simulink model "second"  (R2024b)
settings: Solver=VariableStepAuto  StartTime=0.0  StopTime=45  RelTol=1e-3
settings Model: Creator=asus  LastModifiedBy=asus
settings HardwareCC: TargetBitPerPointer=64  TargetBitPerSizeT=64  TargetBitPerPtrDiffT=64  TargetLongLongMode=on  TargetIntDivRoundTo=Zero  TargetEndianess=LittleEndian  TargetWordSize=64  TargetHWDeviceType=MATLAB Host  ProdEqTarget=off
settings RTWCC: Description=Rapid Simulation Target  SystemTargetFile=rsim.tlc  TemplateMakefile=rsim_default_tmf
settings RSimTargetCC: TargetLangStandard=C99 (ISO)  InstructionSetFMA=off  OptimizeReductions=off  LogToMDFFile=off

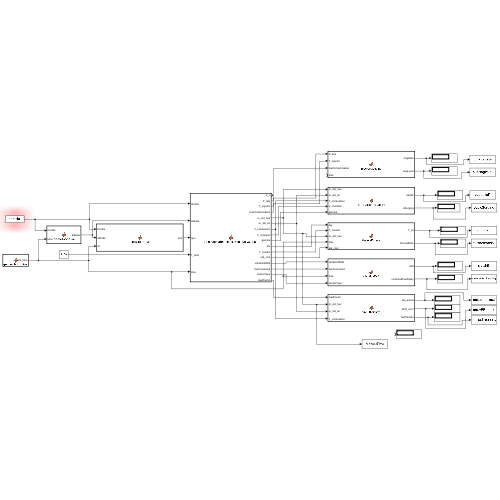
[thumbnail: Simulink's stored preview of the top-level diagram]
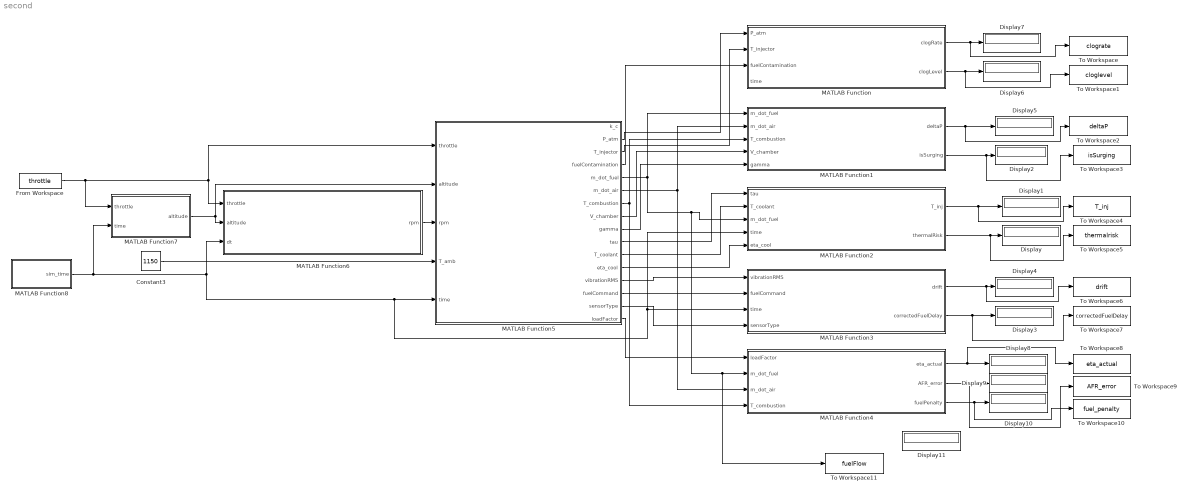
== system second ==
  Constant3 : Constant  Value=1150
  Display{,1..11} (12 alike) : Display
  From Workspace : FromWorkspace  VariableName=throttle
  MATLAB Function : MATLAB Function  TreatAsAtomicUnit=on
  MATLAB Function1 : MATLAB Function  TreatAsAtomicUnit=on
  MATLAB Function2 : MATLAB Function  TreatAsAtomicUnit=on
  MATLAB Function3 : MATLAB Function  TreatAsAtomicUnit=on
  MATLAB Function4 : MATLAB Function  TreatAsAtomicUnit=on
  MATLAB Function5 : MATLAB Function  TreatAsAtomicUnit=on
  MATLAB Function6 : MATLAB Function  TreatAsAtomicUnit=on
  MATLAB Function7 : MATLAB Function  TreatAsAtomicUnit=on
  MATLAB Function8 : MATLAB Function  TreatAsAtomicUnit=on
  To Workspace : ToWorkspace  VariableName=clograte  SaveFormat=Timeseries  SampleTime=-1
  To Workspace1 : ToWorkspace  VariableName=cloglevel  SaveFormat=Timeseries  SampleTime=-1
  To Workspace10 : ToWorkspace  VariableName=fuel_penalty  SaveFormat=Timeseries  SampleTime=-1
  To Workspace11 : ToWorkspace  VariableName=fuelFlow  SaveFormat=Timeseries  SampleTime=-1
  To Workspace2 : ToWorkspace  VariableName=deltaP  SaveFormat=Timeseries  SampleTime=-1
  To Workspace3 : ToWorkspace  VariableName=isSurging  SaveFormat=Timeseries  SampleTime=-1
  To Workspace4 : ToWorkspace  VariableName=T_inj  SaveFormat=Timeseries  SampleTime=-1
  To Workspace5 : ToWorkspace  VariableName=thermalrisk  SaveFormat=Timeseries  SampleTime=-1
  To Workspace6 : ToWorkspace  VariableName=drift  SaveFormat=Timeseries  SampleTime=-1
  To Workspace7 : ToWorkspace  VariableName=correctedFuelDelay  SaveFormat=Timeseries  SampleTime=-1
  To Workspace8 : ToWorkspace  VariableName=eta_actual  SaveFormat=Timeseries  SampleTime=-1
  To Workspace9 : ToWorkspace  VariableName=AFR_error  SaveFormat=Timeseries  SampleTime=-1
  wires:
  MATLAB Function6/1(rpm) -> MATLAB Function5/3(rpm)
  From Workspace/1 -> MATLAB Function6/1(throttle), MATLAB Function5/1(throttle), MATLAB Function7/1(throttle)
  MATLAB Function7/1(altitude) -> MATLAB Function5/2(altitude), MATLAB Function6/2(altitude)
  MATLAB Function8/1(sim_time) -> MATLAB Function7/2(time), MATLAB Function3/3(time), MATLAB Function2/4(time), MATLAB Function5/5(time), MATLAB Function6/3(dt)
  MATLAB Function5/4(fuelContamination) -> MATLAB Function/3(fuelContamination)
  MATLAB Function5/3(T_injector) -> MATLAB Function/2(T_injector)
  MATLAB Function5/2(P_atm) -> MATLAB Function/1(P_atm)
  MATLAB Function5/5(m_dot_fuel) -> MATLAB Function2/3(m_dot_fuel), To Workspace11/1, MATLAB Function4/2(m_dot_fuel), MATLAB Function1/1(m_dot_fuel)
  MATLAB Function5/6(m_dot_air) -> MATLAB Function4/3(m_dot_air), MATLAB Function1/2(m_dot_air)
  MATLAB Function5/7(T_combustion) -> MATLAB Function4/4(T_combustion), MATLAB Function1/3(T_combustion)
  MATLAB Function5/8(V_chamber) -> MATLAB Function1/4(V_chamber)
  MATLAB Function5/9(gamma) -> MATLAB Function1/5(gamma)
  MATLAB Function5/10(tau) -> MATLAB Function2/1(tau)
  MATLAB Function5/11(T_coolant) -> MATLAB Function2/2(T_coolant)
  MATLAB Function5/12(eta_cool) -> MATLAB Function2/5(eta_cool)
  MATLAB Function5/13(vibrationRMS) -> MATLAB Function3/1(vibrationRMS)
  MATLAB Function5/14(fuelCommand) -> MATLAB Function3/2(fuelCommand)
  MATLAB Function5/15(sensorType) -> MATLAB Function3/4(sensorType)
  MATLAB Function5/16(loadFactor) -> MATLAB Function4/1(loadFactor)
  Constant3/1 -> MATLAB Function5/4(T_amb)
  MATLAB Function2/2(thermalRisk) -> To Workspace5/1, Display/1
  MATLAB Function2/1(T_inj) -> To Workspace4/1, Display1/1
  MATLAB Function1/2(isSurging) -> To Workspace3/1, Display2/1
  MATLAB Function/1(clogRate) -> To Workspace/1, Display7/1
  MATLAB Function1/1(deltaP) -> To Workspace2/1, Display5/1
  MATLAB Function3/1(drift) -> To Workspace6/1, Display4/1
  MATLAB Function3/2(correctedFuelDelay) -> To Workspace7/1, Display3/1
  MATLAB Function4/2(AFR_error) -> To Workspace9/1, Display9/1
  MATLAB Function4/1(eta_actual) -> To Workspace8/1, Display8/1
  MATLAB Function4/3(fuelPenalty) -> To Workspace10/1, Display10/1
  MATLAB Function/2(clogLevel) -> To Workspace1/1, Display6/1

== matlab function second/MATLAB Function6 ==
  data: throttle input; rpm output; altitude input; dt input
function rpm = calculateRPM(throttle, altitude, dt)
    %#codegen
    
    % Input validation for Simulink and codegen
    coder.inline('always'); % Inline the function for efficiency
    assert(isscalar(throttle) && isreal(throttle) && throttle >= 0 && throttle <= 1, ...
           'Throttle must be a scalar in [0, 1]');
    assert(isscalar(altitude) && isreal(altitude) && altitude >= 0, ...
           'Altitude must be a non-negative scalar');
    assert(isscalar(dt) && isreal(dt) && dt > 0, ...
           'Time step (dt) must be a positive scalar');
    
    % Initialize persistent variable for RPM history
    persistent rpm_prev
    if isempty(rpm_prev)
        rpm_prev = 800.0; % Engine idle speed (double)
    end
    
    % Basic RPM calculation
    base_rpm = 800.0 + (throttle * 4000.0); % Linear throttle response (scaled for realistic RPM)
    altitude_factor = max(0.5, 1.0 - (altitude / 15000.0)); % Altitude compensation
    
    % Apply first-order lag to simulate engine response
    target_rpm = base_rpm * altitude_factor;
    time_constant = 2.0; % Seconds for 63% response
    rpm = rpm_prev + (target_rpm - rpm_prev) * (dt / time_constant);
    
    % Ensure RPM stays within realistic bounds
    rpm = min(max(rpm, 800.0), 6000.0); % Bound RPM between idle (800) and max (6000)
    
    % Store current RPM for next iteration
    rpm_prev = rpm;
    
    % Ensure output is scalar double
    rpm = double(rpm);
end

== matlab function second/MATLAB Function7 ==
  data: throttle input; altitude output; time input
function altitude = throttleToAltitude(throttle, time)
    % Constants
    max_thrust = 50000;   % N (adjust per helicopter)
    m = 3000;             % kg
    g = 9.81;             % m/s²
    k = 1.3;              % Drag factor
    
    % Thrust calculation
    T = (throttle/100) * max_thrust;
    
    % Vertical acceleration
    dh_dt = (T - m*g) / (m*k);
    
    % Integrate to get altitude
    persistent alt_prev;
    if isempty(alt_prev)
        alt_prev = 0;  % Start at ground level
    end
    altitude = alt_prev + dh_dt * time;
    altitude = max(0, altitude);  % No negative altitude
    alt_prev = altitude;
end

== matlab function second/MATLAB Function8 ==
  data: sim_time output
function sim_time = getSimulationTime()
    persistent start_time;
    if isempty(start_time)
        start_time = posixtime(datetime('now'));  % Unix timestamp at start
    end
    sim_time = posixtime(datetime('now')) - start_time;  % Elapsed seconds
end

== matlab function second/MATLAB Function1 ==
  data: m_dot_fuel input; deltaP output; m_dot_air input; T_combustion input; V_chamber input; isSurging output; gamma input
function [deltaP, isSurging] = combustionInstability(m_dot_fuel, m_dot_air, T_combustion, V_chamber, gamma)
    % Inputs:
    %   m_dot_fuel (kg/s): Fuel mass flow rate
    %   m_dot_air (kg/s): Air mass flow rate
    %   T_combustion (K): Combustion temperature
    %   V_chamber (m³): Combustion chamber volume
    %   gamma: Specific heat ratio (e.g., 1.4 for air)
    
    % Constants
    R = 287;  % Gas constant for air (J/kg·K)
    surgeThreshold = 0.3;  % Threshold for surge detection (empirical)
    
    % Pressure oscillation amplitude (simplified model)
    FAR_actual = m_dot_fuel / m_dot_air;
    FAR_stoich = 0.068;  % Stoichiometric FAR for kerosene-air
    deltaP = sqrt(gamma * R * T_combustion / V_chamber) * abs(FAR_actual - FAR_stoich);
    
    % Surging detection (boolean)
    isSurging = (deltaP > surgeThreshold);
end

== matlab function second/MATLAB Function ==
  data: P_atm input; clogRate output; T_injector input; fuelContamination input; time input; clogLevel output
function [clogRate, clogLevel] = injectorClogging(P_atm, T_injector, fuelContamination, time)
    % Inputs:
    %   P_atm (Pa): Ambient pressure (altitude-dependent)
    %   T_injector (K): Injector temperature
    %   fuelContamination (0-1): Fuel impurity level
    %   time (s): Simulation time (for integration)
    
    % Constants
    P_ref = 101325;     % Reference pressure (Pa, sea level)
    R = 8.314;          % Universal gas constant
    E_a = 50000;        % Activation energy (J/mol, empirical)
    k_c = 0.001;        % Empirical clogging rate constant
    
    % Clogging rate (dC/dt)
    clogRate = k_c * (P_atm / P_ref) * exp(-E_a / (R * T_injector)) * fuelContamination;
    
    % Clog level (integrate rate over time)
    persistent cumulativeClog;
    if isempty(cumulativeClog)
        cumulativeClog = 0;
    end
    cumulativeClog = cumulativeClog + clogRate * time;
    clogLevel = min(cumulativeClog, 100);  % Cap at 100%
end

== matlab function second/MATLAB Function2 ==
  data: tau input; T_coolant input; m_dot_fuel input; T_inj output; time input; thermalRisk output; eta_cool input
function [T_inj, thermalRisk] = thermalStress(tau, T_coolant, m_dot_fuel, time, eta_cool)
    %#codegen
    % Constants
    T_max = 500;          % Max allowable injector temp (K)
    k_heat = 0.05;        % Heat gain coefficient
    k_cool = 0.1;         % Cooling coefficient
    
    % 1. Heat generation (always >= 0)
    Q_gen = max(0, k_heat * abs(tau) * abs(m_dot_fuel));
    
    % 2. Heat dissipation (always >= 0)
    Q_cool = max(0, k_cool * abs(eta_cool) * (T_coolant - 298));
    
    % 3. Temperature calculation (Euler integration)
    persistent T_inj_prev;
    if isempty(T_inj_prev)
        T_inj_prev = T_coolant;  % Initialize to coolant temp
    end
    T_inj = T_inj_prev + (Q_gen - Q_cool) * time;
    T_inj = max(T_coolant, T_inj);  % Never below coolant temp
    T_inj_prev = T_inj;
    
    % 4. Non-negative thermal risk (0-1 scale)
    thermalRisk = max(0, min(1, (T_inj - 0.7*T_max)/(0.3*T_max)));
end

== matlab function second/MATLAB Function3 ==
  data: vibrationRMS input; fuelCommand input; time input; sensorType input; drift output; correctedFuelDelay output
function [drift, correctedFuelDelay] = vibrationDrift(vibrationRMS, fuelCommand, time, sensorType)
    % Inputs:
    %   vibrationRMS (m/s²): Vibration magnitude (RMS)
    %   fuelCommand (kg/s): Commanded fuel flow rate
    %   time (s): Simulation time
    %   sensorType: 1=Pressure, 2=Temperature (different drift behaviors)
    
    % Constants
    kBias = 0.02;       % Drift coefficient (empirical)
    kPhase = 1e-4;      % Phase delay coefficient
    maxDrift = 0.15;    % 15% max error
    
    % 1. Sensor Bias Drift (DC offset)
    drift = kBias * vibrationRMS * time;
    drift = min(drift, maxDrift);  % Clamp drift
    
    % 2. Fuel Delivery Delay (phase lag)
    if sensorType == 1
        % Pressure sensor: Delay ~ vibration^2
        phaseLag = kPhase * (vibrationRMS^2) * fuelCommand;
    else
        % Temperature sensor: Delay ~ linear
        phaseLag = kPhase * vibrationRMS * fuelCommand;
    end
    
    % Compensated delay (example: subtract estimated lag)
    correctedFuelDelay = max(0, fuelCommand - phaseLag);
end

== matlab function second/MATLAB Function4 ==
  data: loadFactor input; m_dot_fuel input; m_dot_air input; T_combustion input; eta_actual output; AFR_error output; fuelPenalty output
function [eta_actual, AFR_error, fuelPenalty] = fuelEfficiency(loadFactor, m_dot_fuel, m_dot_air, T_combustion)
    % Inputs:
    %   loadFactor (0-1): Current load / Rated load
    %   m_dot_fuel (kg/s): Fuel mass flow rate
    %   m_dot_air (kg/s): Air mass flow rate
    %   T_combustion (K): Combustion chamber temperature
    
    % Constants
    AFR_stoich = 14.7;       % Stoichiometric AFR for kerosene
    AFR_opt_map = [12.5, 14.7, 16.3];  % Optimal AFR at [0.3, 0.7, 1.0] loadFactor
    
    % 1. Interpolate optimal AFR for current load
    loadPoints = [0.3, 0.7, 1.0];
    AFR_opt = interp1(loadPoints, AFR_opt_map, loadFactor, 'pchip');
    
    % 2. Calculate actual AFR and error
    AFR_actual = m_dot_air / max(m_dot_fuel, 1e-6);  % Avoid division by zero
    AFR_error = AFR_actual - AFR_opt;
    
    % 3. Efficiency penalty (0-1 scale)
    T_norm = T_combustion / 1000;  % Normalized temperature
    fuelPenalty = exp(-0.5 * (AFR_error^2)) * (1 - 0.2 * loadFactor * T_norm);
    eta_actual = 0.95 * fuelPenalty;  % Baseline 95% efficiency scaled by penalty
end

== matlab function second/MATLAB Function5 ==
  data: throttle input; k_c output; altitude input; rpm input; T_amb input; P_atm output; time input; T_injector output; fuelContamination output; m_dot_fuel output; m_dot_air output; T_combustion output; V_chamber output; gamma output; tau output; T_coolant output; eta_cool output; vibrationRMS output; fuelCommand output; sensorType output; loadFactor output
function [k_c, P_atm, T_injector, fuelContamination, ...
          m_dot_fuel, m_dot_air, T_combustion, V_chamber, gamma, ...
          tau, T_coolant, eta_cool, ...
          vibrationRMS, fuelCommand, sensorType, ...
          loadFactor] = ...
          generateFailureInputs_SeparateOutputs(throttle, altitude, rpm, T_amb, time)
% Inputs:
%   throttle (0-100%) : Throttle position
%   altitude (m)      : Current altitude
%   rpm               : Engine RPM
%   T_amb (°C)        : Ambient temperature
%   time (s)          : Simulation time
%
% Outputs:
%   All parameters split into individual variables (no structs)

%% 1. Derived Intermediate Variables
P_atm = 101325 * exp(-altitude / 8500);    % Atmospheric pressure (Pa)
T_comb = 300 + 0.6 * throttle + 0.01 * rpm; % Combustion temp (K)
torque = (throttle / 100) * (rpm / 2000);  % Normalized torque (0-1)
fuelFlow = 0.02 * throttle * sqrt(abs(rpm));     % Fuel flow rate (kg/s)
vibrationRMS = 2 + 0.05 * rpm + 0.1 * (altitude / 1000); % Vibration (m/s²)

%% 2. Injector Clogging Parameters (Failure Mode 1)
k_c = 0.001;                    % Clogging rate constant
T_injector = T_comb - 50;       % Injector temp (K)
fuelContamination = 0.1 + 0.01 * (time / 3600); % Degrades over time

%% 3. Combustion Instability Parameters (Failure Mode 2)
m_dot_fuel = fuelFlow;
m_dot_air = fuelFlow * 14.7;    % Assume stoichiometric AFR
T_combustion = T_comb;
V_chamber = 0.002;              % Combustion chamber volume (m³)
gamma = 1.4;                    % Specific heat ratio

%% 4. Heat Management Parameters (Failure Mode 3)
tau = torque * 500;             % Torque (Nm) scaled
T_coolant = T_amb + 10 + 0.2 * throttle; % Coolant temp (°C)
eta_cool = 0.9 - 0.001 * time;  % Cooling efficiency degrades

%% 5. Vibration Drift Parameters (Failure Mode 4)
fuelCommand = fuelFlow;
sensorType = 1;                 % 1=Pressure, 2=Temperature

%% 6. Fuel Inefficiency Parameters (Failure Mode 5)
loadFactor = torque;            % Normalized load (0-1)
end
